simulink model "adc_demo"  (R2020a)
settings: Solver=VariableStepDiscrete  StartTime=0.0  StopTime=1  RelTol=1e-3  EnableMultiTasking=on
libraries: simulink_extras x3, dspstat3 x1
settings Model: Creator=rcheng  LastModifiedBy=Adriana
settings DataIOCC: LimitDataPoints=on  SaveFormat=Array  SignalLoggingSaveFormat=ModelDataLogs  ReturnWorkspaceOutputs=off
settings OptimizationCC: ExpressionDepthLimit=2147483647  InitFltsAndDblsToZero=on  LifeSpan=inf
settings DebuggingCC: UnderspecifiedInitializationDetection=Classic  MergeDetectMultiDrivingBlocksExec=none  SolverPrmCheckMsg=warning  FcnCallInpInsideContextMsg=warning  StateNameClashWarn=warning  SFUnexpectedBacktrackingDiag=warning  SFNoUnconditionalDefaultTransitionDiag=warning  SFExecutionAtInitializationDiag=none  ArithmeticOperatorsInVariantConditions=warning
settings HardwareCC: ProdBitPerPointer=32  ProdBitPerSizeT=32  ProdBitPerPtrDiffT=32  ProdLargestAtomicFloat=None  ProdIntDivRoundTo=Undefined  ProdEndianess=Unspecified  ProdWordSize=32  ProdHWDeviceType=32-bit Generic
settings ModelReferenceCC: PropagateSignalLabelsOutOfModel=off
settings SFSimCC: SimUseLocalCustomCode=off  CustomCodeUndefinedFunction=UseInterfaceOnly
settings RTWCC: RTWUseLocalCustomCode=off
settings CodeAppCC: StateflowObjectComments=on
settings GRTTargetCC: TargetLangStandard=C89/C90 (ANSI)  CombineOutputUpdateFcns=off  GRTInterface=on
settings ConfigComp: CovMetricSettings=dw  CovSaveCumulativeToWorkspaceVar=on  CovSaveSingleToWorkspaceVar=on  CovExternalEMLEnable=off  CovSFcnEnable=off

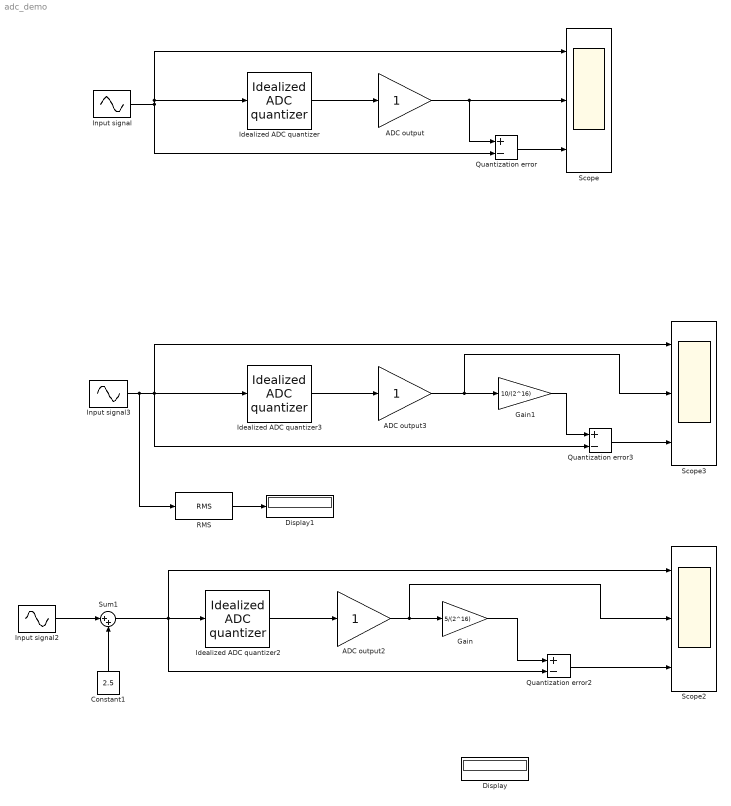
== system adc_demo ==
  ADC output : Gain
  ADC output2 : Gain
  ADC output3 : Gain
  Constant1 : Constant  Value=2.5
  Display : Display
  Display1 : Display
  Gain : Gain  Gain=5/(2^16)
  Gain1 : Gain  Gain=10/(2^16)
  Idealized ADC quantizer : simulink_extras/Additional Discrete/Idealized ADC quantizer  NumberOfConverterBits=16  Vmin=0  Vmax=5  OutputDataType=int16  OutputNegativeValues=on
  Idealized ADC quantizer2 : simulink_extras/Additional Discrete/Idealized ADC quantizer  NumberOfConverterBits=16  Vmin=0  Vmax=5  OutputDataType=uint16  OutputNegativeValues=on
  Idealized ADC quantizer3 : simulink_extras/Additional Discrete/Idealized ADC quantizer  NumberOfConverterBits=16  Vmin=-5  Vmax=5  OutputDataType=int16  OutputNegativeValues=on
  Input signal : Sin  Amplitude=2.5  Frequency=2*pi*100  SampleTime=1/10000
  Input signal2 : Sin  Amplitude=2.5  Frequency=2*pi*100  SampleTime=1/10000
  Input signal3 : Sin  Amplitude=2.5  Frequency=2*pi*100  SampleTime=1/10000
  Quantization error : Sum  Inputs=+-
  Quantization error2 : Sum  Inputs=+-
  Quantization error3 : Sum  Inputs=+-
  RMS : dspstat3/RMS  run=off  directionMode=Entire input  dimension=1  InputProcessing=Columns as channels (frame based)  reset_popup=None
  Scope : Scope  NumInputPorts=3
  Scope2 : Scope  NumInputPorts=3
  Scope3 : Scope  NumInputPorts=3
  Sum1 : Sum  Inputs=|++
  wires:
  Quantization error/1 -> Scope/3
  Idealized ADC quantizer/1 -> ADC output/1
  ADC output/1 -> Quantization error/1, Scope/2
  Input signal/1 -> Idealized ADC quantizer/1, Scope/1, Quantization error/2
  Idealized ADC quantizer2/1 -> ADC output2/1
  Sum1/1 -> Quantization error2/2, Idealized ADC quantizer2/1, Scope2/1
  Input signal2/1 -> Sum1/1
  Quantization error2/1 -> Scope2/3
  Quantization error3/1 -> Scope3/3
  ADC output3/1 -> Scope3/2, Gain1/1
  Idealized ADC quantizer3/1 -> ADC output3/1
  Input signal3/1 -> RMS/1, Quantization error3/2, Idealized ADC quantizer3/1, Scope3/1
  ADC output2/1 -> Scope2/2, Gain/1
  Constant1/1 -> Sum1/2
  Gain/1 -> Quantization error2/1
  Gain1/1 -> Quantization error3/1
  RMS/1 -> Display1/1
